simulink library "lib_transformations"  (Simulink 9.0)
settings: Solver=ode45  StartTime=0.0  StopTime=10.0  RelTol=1e-3  EnableMultiTasking=on
undefined symbols (not defined in the file or in its folder): r_i_B_C
settings Model: SuppressorTable=22 serialization::archive 11 0 6 0 0 0 11 0  Creator=schappler  LastModifiedBy=schappler

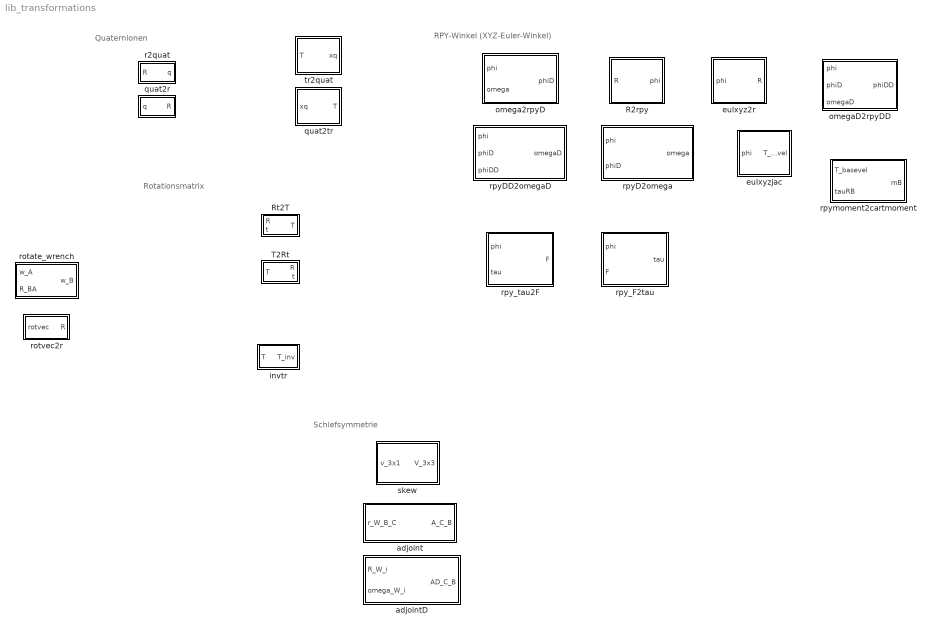
== system lib_transformations ==
  note: Schiefsymmetrie
  note: Rotationsmatrix
  note: Quaternionen
  note: RPY-Winkel (XYZ-Euler-Winkel)
  R2rpy : Subsystem
  Rt2T : Subsystem
  T2Rt : Subsystem
  adjoint : Subsystem  mask{KSName_W='W', PktName_B='B', PktName_C='C'}
      mask prompts: KSName_W "KSName_W: Name des Bezugs-Koordinatensystems W (nur für Block-Beschriftung)"; PktName_B "PktName_B: Name des Punktes B (nur für Block-Beschriftung)"; PktName_C "PktName_C: Name des Punktes C (nur für Block-Beschriftung)"
      mask help: Adjunkt-Matrix. Siehe Funktion adjoint_jacobian
      mask Display:
      | port_label('input', 1, sprintf('_{(%s)}r_{%s,%s}', KSName_W, PktName_B, PktName_C), 'texmode', 'on')
      | port_label('output', 1, sprintf('_{(%s)}A(%s,%s)', KSName_W, PktName_C, PktName_B), 'texmode', 'on')
  adjointD : Subsystem  mask{r_i_B_C=r_i_B_C, KSName_W='W', KSName_i='i', PktName_B='B', PktName_C='C'}
      mask prompts: r_i_B_C "r_i_B_C: Vektor vom Punkt B zum Punkt C ausgedrückt im KS i"; KSName_W "KSName_W: Name des Bezugs-Koordinatensystems W (nur für Block-Beschriftung)"; KSName_i "KSName_i: Name des Koordinatensystems i (nur für Block-Beschriftung)"; PktName_B "PktName_B: Name des Punktes B (nur für Block-Beschriftung)"; PktName_C "PktName_C: Name des Punktes C (nur für Block-Beschriftung)"
      mask help: Zeitableitung der Adjunkt-Matrix. Siehe Funktion adjointD_jacobian
      mask Display:
      | port_label('input', 1, sprintf('_{(%s)}\\omega_{%s,%s}', KSName_W, KSName_W, KSName_i), 'texmode', 'on')
      | port_label('input', 2, sprintf('^{%s}R_%s', KSName_W, KSName_i), 'texmode', 'on')
      | 
      | port_label('output', 1, sprintf('_{(%s)}AD(%s,%s)', KSName_W, PktName_C, PktName_B), 'texmode', 'on')
  eulxyzjac : Subsystem
  invtr : Subsystem
  omega2rpyD : Subsystem
  omegaD2rpyDD : Subsystem
  quat2r : Subsystem
  quat2tr : Subsystem
  r2quat : Subsystem
  rotate_wrench : Subsystem  mask{Name_A='A', Name_B='B'}
      mask prompts: Name_A "Name KS A (nur für Beschriftung)"; Name_B "Name KS B (nur für Beschriftung)"
      mask Display:
      | port_label('input', 1, sprintf('_{(%s)}w', Name_A), 'texmode', 'on')
      | port_label('input', 2, sprintf('^{(%s)}R_{(%s)}', Name_B, Name_A), 'texmode', 'on')
      | port_label('output', 1, sprintf('_{(%s)}w', Name_B), 'texmode', 'on')
  rotvec2r : Subsystem
  eulxyz2r : Subsystem
  rpyD2omega : Subsystem
  rpyDD2omegaD : Subsystem
  rpy_F2tau : Subsystem
  rpy_tau2F : Subsystem
  rpymoment2cartmoment : Subsystem
  skew : Subsystem
  tr2quat : Subsystem

== system lib_transformations/R2rpy ==
  R : Inport  PortDimensions=[3 3]
  R2rpy : MATLAB Function  TreatAsAtomicUnit=on
  phi : Outport  PortDimensions=3
  wires:
  R/1 -> R2rpy/1(R)
  R2rpy/1(phi) -> phi/1

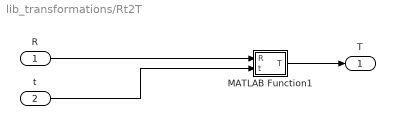
== system lib_transformations/Rt2T ==
  R : Inport  PortDimensions=[3 3]
  t : Inport  Port=2  PortDimensions=3
  MATLAB Function1 : MATLAB Function  TreatAsAtomicUnit=on
  T : Outport  PortDimensions=[4 4]
  wires:
  MATLAB Function1/1(T) -> T/1
  R/1 -> MATLAB Function1/1(R)
  t/1 -> MATLAB Function1/2(t)

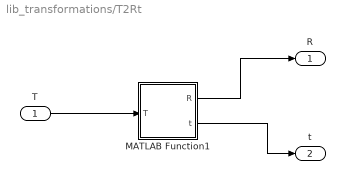
== system lib_transformations/T2Rt ==
  T : Inport  PortDimensions=[4 4]
  MATLAB Function1 : MATLAB Function  TreatAsAtomicUnit=on
  R : Outport  PortDimensions=[3 3]
  t : Outport  Port=2  PortDimensions=3
  wires:
  MATLAB Function1/1(R) -> R/1
  T/1 -> MATLAB Function1/1(T)
  MATLAB Function1/2(t) -> t/1

== system lib_transformations/adjoint ==
  r_W_B_C : Inport  PortDimensions=3
  adjoint_fcn : MATLAB Function  TreatAsAtomicUnit=on
  A_C_B : Outport  PortDimensions=[6 6]
  wires:
  r_W_B_C/1 -> adjoint_fcn/1(r_B_C)
  adjoint_fcn/1(A_C_B) -> A_C_B/1

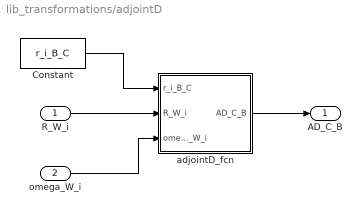
== system lib_transformations/adjointD ==
  R_W_i : Inport  PortDimensions=[3 3]
  omega_W_i : Inport  Port=2  PortDimensions=3
  Constant : Constant  Value=r_i_B_C
  adjointD_fcn : MATLAB Function  TreatAsAtomicUnit=on
  AD_C_B : Outport  PortDimensions=[6 6]
  wires:
  Constant/1 -> adjointD_fcn/1(r_i_B_C)
  adjointD_fcn/1(AD_C_B) -> AD_C_B/1
  R_W_i/1 -> adjointD_fcn/2(R_W_i)
  omega_W_i/1 -> adjointD_fcn/3(omega_W_i)

== system lib_transformations/eulxyzjac ==
  phi : Inport  PortDimensions=3
  eulxyzjac_Fcn : MATLAB Function  TreatAsAtomicUnit=on
  T_angvel : Outport  PortDimensions=[3 3]
  wires:
  phi/1 -> eulxyzjac_Fcn/1(phi)
  eulxyzjac_Fcn/1(T_angvel) -> T_angvel/1

== system lib_transformations/invtr ==
  T : Inport
  invtr : MATLAB Function  TreatAsAtomicUnit=on
  T_inv : Outport
  wires:
  invtr/1(T_inv) -> T_inv/1
  T/1 -> invtr/1(T)

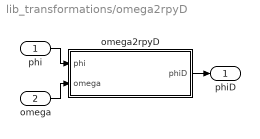
== system lib_transformations/omega2rpyD ==
  phi : Inport  PortDimensions=3
  omega : Inport  Port=2  PortDimensions=3
  omega2rpyD : MATLAB Function  TreatAsAtomicUnit=on
  phiD : Outport  PortDimensions=3
  wires:
  phi/1 -> omega2rpyD/1(phi)
  omega/1 -> omega2rpyD/2(omega)
  omega2rpyD/1(phiD) -> phiD/1

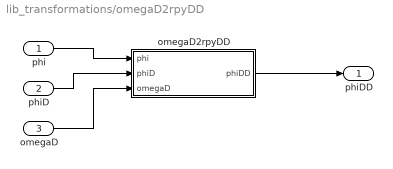
== system lib_transformations/omegaD2rpyDD ==
  phi : Inport  PortDimensions=3
  phiD : Inport  Port=2  PortDimensions=3
  omegaD : Inport  Port=3  PortDimensions=3
  omegaD2rpyDD : MATLAB Function  TreatAsAtomicUnit=on
  phiDD : Outport  PortDimensions=3
  wires:
  phi/1 -> omegaD2rpyDD/1(phi)
  omegaD/1 -> omegaD2rpyDD/3(omegaD)
  omegaD2rpyDD/1(phiDD) -> phiDD/1
  phiD/1 -> omegaD2rpyDD/2(phiD)

== system lib_transformations/quat2r ==
  q : Inport  PortDimensions=4
  MATLAB Function1 : MATLAB Function  TreatAsAtomicUnit=on
  R : Outport  PortDimensions=[3 3]
  wires:
  MATLAB Function1/1(R) -> R/1
  q/1 -> MATLAB Function1/1(q)

== system lib_transformations/quat2tr ==
  xq : Inport  PortDimensions=[1 7]
  quat2tr : MATLAB Function  TreatAsAtomicUnit=on
  T : Outport  PortDimensions=[4 4]
  wires:
  xq/1 -> quat2tr/1(xq)
  quat2tr/1(T) -> T/1

== system lib_transformations/r2quat ==
  R : Inport  PortDimensions=[3 3]
  MATLAB Function1 : MATLAB Function  TreatAsAtomicUnit=on
  q : Outport  PortDimensions=4
  wires:
  MATLAB Function1/1(q) -> q/1
  R/1 -> MATLAB Function1/1(R)

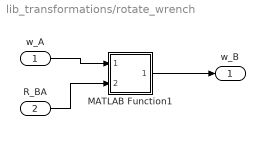
== system lib_transformations/rotate_wrench ==
  w_A : Inport  PortDimensions=6
  R_BA : Inport  Port=2  PortDimensions=[3 3]
  MATLAB Function1 : MATLAB Function  TreatAsAtomicUnit=on
  w_B : Outport  PortDimensions=6
  wires:
  w_A/1 -> MATLAB Function1/1(w_A)
  MATLAB Function1/1(w_B) -> w_B/1
  R_BA/1 -> MATLAB Function1/2(R_BA)

== system lib_transformations/rotvec2r ==
  rotvec : Inport
  rotvec2r : MATLAB Function  TreatAsAtomicUnit=on
  R : Outport
  wires:
  rotvec2r/1(R) -> R/1
  rotvec/1 -> rotvec2r/1(rotvec)

== system lib_transformations/eulxyz2r ==
  phi : Inport
  rpy2R : MATLAB Function  TreatAsAtomicUnit=on
  R : Outport
  wires:
  phi/1 -> rpy2R/1(phi)
  rpy2R/1(R) -> R/1

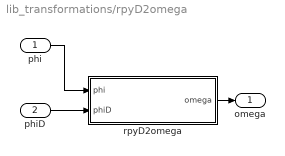
== system lib_transformations/rpyD2omega ==
  phi : Inport
  phiD : Inport  Port=2
  rpyD2omega : MATLAB Function  TreatAsAtomicUnit=on
  omega : Outport  PortDimensions=3
  wires:
  phi/1 -> rpyD2omega/1(phi)
  phiD/1 -> rpyD2omega/2(phiD)
  rpyD2omega/1(omega) -> omega/1

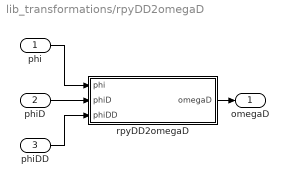
== system lib_transformations/rpyDD2omegaD ==
  phi : Inport
  phiD : Inport  Port=2
  phiDD : Inport  Port=3
  rpyDD2omegaD : MATLAB Function  TreatAsAtomicUnit=on
  omegaD : Outport  PortDimensions=3
  wires:
  phi/1 -> rpyDD2omegaD/1(phi)
  phiD/1 -> rpyDD2omegaD/2(phiD)
  rpyDD2omegaD/1(omegaD) -> omegaD/1
  phiDD/1 -> rpyDD2omegaD/3(phiDD)

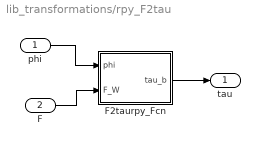
== system lib_transformations/rpy_F2tau ==
  phi : Inport  PortDimensions=3
  F : Inport  Port=2  PortDimensions=6
  F2taurpy_Fcn : MATLAB Function  TreatAsAtomicUnit=on
  tau : Outport  PortDimensions=6
  wires:
  F/1 -> F2taurpy_Fcn/2(F_W)
  F2taurpy_Fcn/1(tau_b) -> tau/1
  phi/1 -> F2taurpy_Fcn/1(phi)

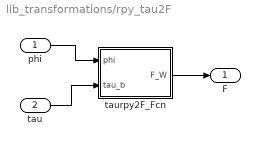
== system lib_transformations/rpy_tau2F ==
  phi : Inport  PortDimensions=3
  tau : Inport  Port=2  PortDimensions=6
  taurpy2F_Fcn : MATLAB Function  TreatAsAtomicUnit=on
  F : Outport  PortDimensions=6
  wires:
  tau/1 -> taurpy2F_Fcn/2(tau_b)
  taurpy2F_Fcn/1(F_W) -> F/1
  phi/1 -> taurpy2F_Fcn/1(phi)

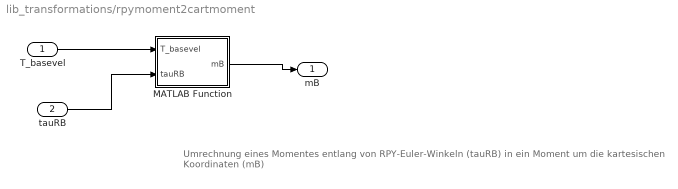
== system lib_transformations/rpymoment2cartmoment ==
  note: Umrechnung eines Momentes entlang von RPY-Euler-Winkeln (tauRB) in ein Moment um die kartesischen Koordinaten (mB)
  T_basevel : Inport  PortDimensions=[3 3]
  tauRB : Inport  Port=2  PortDimensions=3
  MATLAB Function : MATLAB Function  TreatAsAtomicUnit=on
  mB : Outport  PortDimensions=3
  wires:
  T_basevel/1 -> MATLAB Function/1(T_basevel)
  MATLAB Function/1(mB) -> mB/1
  tauRB/1 -> MATLAB Function/2(tauRB)

== system lib_transformations/skew ==
  v_3x1 : Inport
  skew_fcn : MATLAB Function  TreatAsAtomicUnit=on
  V_3x3 : Outport
  wires:
  v_3x1/1 -> skew_fcn/1(v)
  skew_fcn/1(V) -> V_3x3/1

== system lib_transformations/tr2quat ==
  T : Inport  PortDimensions=[4 4]
  tr2quat : MATLAB Function  TreatAsAtomicUnit=on
  xq : Outport  PortDimensions=7
  wires:
  T/1 -> tr2quat/1(T)
  tr2quat/1(xq) -> xq/1

== matlab function quat2r/MATLAB Function1 ==
  data: R output double; q input double
function R = quat2r(q)
%#codegen

R = quat2r(q);

== matlab function tr2quat/tr2quat ==
  data: T input double; xq output double
function xq = tr2quat(T)
%#codegen

xq = tr2quat(T);

== matlab function r2quat/MATLAB Function1 ==
  data: R input double; q output double
function q = r2quat(R)
%#codegen

q = r2quat(R)';

== matlab function rotate_wrench/MATLAB Function1 ==
  data: w_B output double; w_A input double; R_BA input double
% Rotiere 6x1-Vektor mit Kraftwinde (wrench) oder allgemeine
% Geschwindingkeit (twist) in ein anderes Koordinatensystem
% 
% Input:
% w_A
%   Vektor in KS A
% R_BA
%   Rotationsmatrix von A nach B
% 
% Output:
% w_B
%   Vektor in KS b

% Moritz Schappler, schappler@irt.uni-hannover.de, 2015-09
% (c) Institut für Regelungstechnik, Universität Hannover

function w_B = rotate_wrench(w_A, R_BA)
%#codegen

w_B = rotate_wrench(w_A, R_BA);

== matlab function Rt2T/MATLAB Function1 ==
  data: R input double; T output double; t input double
function T = rt2t(R,t)
%#codegen
assert(isa(R,'double') && isreal(R) && all(size(R) == [3 3]));
assert(isa(t,'double') && isreal(t) && all(size(t) == [3 1]));
T = [R, t; [0 0 0 1]];

== matlab function rotvec2r/rotvec2r ==
  data: rotvec input double; R output double
% Rotationsvektor in Rotationsmatrix umrechnen
% 
% Eingang:
% rotvec
%   Rotationsvektor (Achse der Achse-Winkel-Konvention mit Winkel
%   multipliziert)
% 
% Ausgang:
% R
%   Rotationsmatrix

% Moritz Schappler, schappler@irt.uni-hannover.de, 2015-10
% (c) Institut für Regelungstechnik, Universität Hannover

function R = rotvec2r(rotvec)
%% Init
%#codegen
assert(isa(rotvec,'double') && isreal(rotvec) && all(size(rotvec) == [3 1]), ...
  'Rotationsvektor muss [3x1] double sein.');

R = rotvec2r(rotvec);

== matlab function eulxyz2r/rpy2R ==
  data: phi input double; R output double
% RPY-Winkelkonvention in Rotationsmatrix umwandeln
% 
% Input:
%  rpy-Winkel [3x1]
%   Definition: R = rotx(rpy(1))*roty(rpy(2))*rotz(rpy(3));
% Output:
% rpy:
% R [3x3]
%   Rotationsmatrix


% Moritz Schappler, schappler@irt.uni-hannover.de, 2016-05
% (c) Institut für Regelungstechnik, Universität Hannover

function R = fcn(phi)
%#codegen
R = eulxyz2r(phi);

== matlab function rpyD2omega/rpyD2omega ==
  data: phi input double; omega output double; phiD input double
% Konvertiere die erste Zeitableitung der Rotationsdarstellung in RPY-Winkeln in
% Drehgeschwindigkeit
% 
% RPY-Winkel: R=rotx(alpha)*roty(beta)*rotz(gamma)
% 
% Eingabe:
% phi [3x1]
%   RPY-Winkel alpha, beta, gamma. Entsprechen zusammen der Rotationsmatrix
%   R_A_B
% phiD [3x1]
%   1. Zeitableitung der RPY-Winkel alpha, beta, gamma
% Ausgabe:
% omega [3x1]
%   Drehgeschwindigkeit (omega_A_B) von KS_B ausgedrückt in KS_A
% 
% Quelle:
% [ZupanSaj2011] Zupan, Eva and Saje, Miran: Integrating rotation from
% angular velocity 

% Moritz Schappler, schappler@irt.uni-hannover.de, 2016-05
% (c) Institut für Regelungstechnik, Universität Hannover


function omega = fcn(phi, phiD)
%#codegen
omega = rpyD2omega(phi, phiD);

== matlab function eulxyzjac/eulxyzjac_Fcn ==
  data: phi input double; T_angvel output double
% Transformation zwischen Winkelgeschwindigkeit und Ableitung der
% Orientierungsdarstellung für RPY-Winkel (=XYZ-Euler-Winkel).
% 
% Input:
%  rpy-Winkel [3x1] 
%   Definition: R = rotx(rpy(1))*roty(rpy(2))*rotz(rpy(3));

% Output:
% T
%   Transformationsmatrix (3x3) zwischen Winkelgeschwindigkeit im
%   Basiskoordinatensystem und den Zeitableitungen der
%   Rotationsdarstellungen


% Moritz Schappler, schappler@irt.uni-hannover.de, 2016-05
% (c) Institut für Regelungstechnik, Universität Hannover

function T_angvel = fcn(phi)
%#codegen
T_angvel = eulxyzjac(phi);

== matlab function omegaD2rpyDD/omegaD2rpyDD ==
  data: phi input double; phiD input double; omegaD input double; phiDD output double
% Umwandlung einer Winkelgeschwindigkeit in die Zeitableitung der
% RPY-Winkel (Euler-XYZ)
% 
% Eingabe:
% phi [3x1]
%   RPY-Winkel alpha, beta, gamma. Entsprechen zusammen der Rotationsmatrix
%   R_A_B
% phiD [3x1]
%   1. Zeitableitung der RPY-Winkel alpha, beta, gamma
% omegaD [3x1]
%   Drehbeschleunigung (omegaD_A_B) von KS_B ausgedrückt in KS_A
% 
% Ausgabe:
% phiDD [3x1]
%   2. Zeitableitung der RPY-Winkel alpha, beta, gamma

% Moritz Schappler, schappler@irt.uni-hannover.de, 2016-06
% (c) Institut für Regelungstechnik, Universität Hannover

function phiDD = fcn(phi, phiD, omegaD)
%#codegen

T_basevel = eulxyzjac(phi);
TD_basevel = eulxyzjacD(phi, phiD);
phiDD = T_basevel \ ( omegaD - TD_basevel*phiD);

== matlab function rpymoment2cartmoment/MATLAB Function ==
  data: T_basevel input double; mB output double; tauRB input double
function mB = fcn(T_basevel, tauRB)
%#codegen
mB =   (T_basevel') \ tauRB;

== matlab function quat2tr/quat2tr ==
  data: T output double; xq input double
function T = quat2tr(xq)
%#codegen

T = quat2tr(xq);

== matlab function rpy_tau2F/taurpy2F_Fcn ==
  data: phi input double; F_W output double; tau_b input double
% Wandle Kräfte in RPY-Koordinaten in Kräfte und Momente in kartesischen
% Koordinaten um
% 
% Eingabe:
% phi
%   Orientierung des Körpers (RPY-Winkel)
% tau_b
%   Kraft und Moment in verallgemeinerten Koordinaten, die an dem Körper
%   angreifen
% 
% Ausgabe:
% F_W [6x]
%   Kraft und Moment (wrench)

% Moritz Schappler, schappler@irt.uni-hannover.de, 2016-11
% (c) Institut für Regelungstechnik, Universität Hannover

function F_W = fcn(phi, tau_b)
%#codegen
T_angvel = eulxyzjac(phi(1), phi(2), phi(3));
% Kraft
f_W = tau_b(1:3);
% Moment
m_W = (T_angvel')\tau_b(4:6);

F_W = [f_W; m_W];

== matlab function T2Rt/MATLAB Function1 ==
  data: R output double; T input double; t output double
function [R, t] = t2rt(T)
%#codegen
assert(isa(T,'double') && isreal(T) && all(size(T) == [4 4]));
R = T(1:3,1:3);
t = T(1:3,4);

== matlab function rpy_F2tau/F2taurpy_Fcn ==
  data: phi input double; F_W input double; tau_b output double
% Wandle Kräfte und Momente in kartesischen Koordinaten in Kräfte und Momente in 
% RPY-Koordinaten um
% 
% Eingabe:
% phi
%   Orientierung des Körpers (RPY-Winkel)
% tau_b
%   Kraft und Moment in verallgemeinerten Koordinaten, die an dem Körper
%   angreifen
% 
% Ausgabe:
% F_W [6x]
%   Kraft und Moment (wrench)

% Moritz Schappler, schappler@irt.uni-hannover.de, 2017-03
% (c) Institut für Regelungstechnik, Universität Hannover

function tau_b = fcn(phi, F_W)
%#codegen
tau_b = NaN(6,1);
T_angvel = angvelotrans_rpy(phi(1), phi(2), phi(3));
% Kraft
tau_b(1:3) = F_W(1:3);
% Moment
tau_b(4:6) = (T_angvel') * F_W(4:6);

== matlab function skew/skew_fcn ==
  data: v input double; V output double
% Gebe die schiefsymmetrische (Kreuzprodukt-) Matrix zu einem Vektor aus

function V = skew(v)
%% Init
%#codegen
assert(isa(v,'double') && isreal(v) && all(size(v) == [3 1]), ...
  'Vektor muss [3x1] double sein.');

%% Berechnung
V = skew(v);

== matlab function invtr/invtr ==
  data: T input double; T_inv output double
function T_inv = invtr(T)
%#codegen

T_inv = invtr(T);

== matlab function rpyDD2omegaD/rpyDD2omegaD ==
  data: phi input double; omegaD output double; phiD input double; phiDD input double
% Konvertiere die zweite Zeitableitung der Rotationsdarstellung in RPY-Winkeln in
% Drehbeschleunigung
% 
% RPY-Winkel: R=rotx(alpha)*roty(beta)*rotz(gamma)
% 
% Eingabe:
% phi [3x1]
%   RPY-Winkel alpha, beta, gamma. Entsprechen zusammen der Rotationsmatrix
%   R_A_B
% phiD [3x1]
%   1. Zeitableitung der RPY-Winkel alpha, beta, gamma
% phiDD [3x1]
%   2. Zeitableitung der RPY-Winkel alpha, beta, gamma
% Ausgabe:
% omegaD [3x1]
%   Drehbeschleunigung (omegaD_A_B) von KS_B ausgedrückt in KS_A
% 
% Quelle:
% [ZupanSaj2011] Zupan, Eva and Saje, Miran: Integrating rotation from
% angular velocity 

% Moritz Schappler, schappler@irt.uni-hannover.de, 2015-09
% (c) Institut für Regelungstechnik, Universität Hannover


function omegaD = fcn(phi, phiD, phiDD)
%#codegen
omegaD = rpyDD2omegaD(phi, phiD, phiDD);

== matlab function omega2rpyD/omega2rpyD ==
  data: phi input double; phiD output double; omega input double
% Umwandlung einer Winkelgeschwindigkeit in die Zeitableitung der
% RPY-Winkel (Euler-XYZ)
% 
% Eingabe:
% phi [3x1]
%   RPY-Winkel: Koordinatentransformation zwischen A und B
% omega [3x1]
%   Winkelgeschwindigkeit eines Koordinatensystems A, ausgedrückt im KS B
% 
% Ausgabe:
% phiD
%   Zeitableitung der RPY-Winkel phi

% Moritz Schappler, schappler@irt.uni-hannover.de, 2016-05
% (c) Institut für Regelungstechnik, Universität Hannover

function phiD = fcn(phi, omega)
%#codegen
T_angvel = eulxyzjac(phi);
phiD = T_angvel \ omega;

== matlab function R2rpy/R2rpy ==
  data: phi output double; R input double
% Rotationsmatrix in RPY-Winkelkonvention umwandeln
% 
% Input:
% R:
%   [3x3] Rotationsmatrix
% 
% Output:
% rpy:
%   [3x1] rpy-Winkel
%   Definition: R = rotx(rpy(1))*roty(rpy(2))*rotz(rpy(3));

% Moritz Schappler, schappler@irt.uni-hannover.de, 2015-08
% (c) Institut für Regelungstechnik, Universität Hannover

function phi = fcn(R)
%#codegen
phi = r2eulxyz(R)';

== matlab function adjoint/adjoint_fcn ==
  data: r_B_C input double; A_C_B output double
function A_C_B = adjoint(r_B_C)
%#codegen
A_C_B = adjoint_jacobian(r_B_C);

== matlab function adjointD/adjointD_fcn ==
  data: r_i_B_C input double; AD_C_B output double; R_W_i input double; omega_W_i input double
function AD_C_B = adjointD(r_i_B_C, R_W_i, omega_W_i)
%#codegen
AD_C_B = adjointD_jacobian(r_i_B_C, R_W_i, omega_W_i);
